simulink model "Plant0"  (R2020b)
settings: Solver=FixedStepAuto  StartTime=0.0  StopTime=5  FixedStep=1e-06  RelTol=1e-3
settings Model: Creator=99714  LastModifiedBy=99714
settings DataIOCC: SaveOutput=off  SaveTime=off

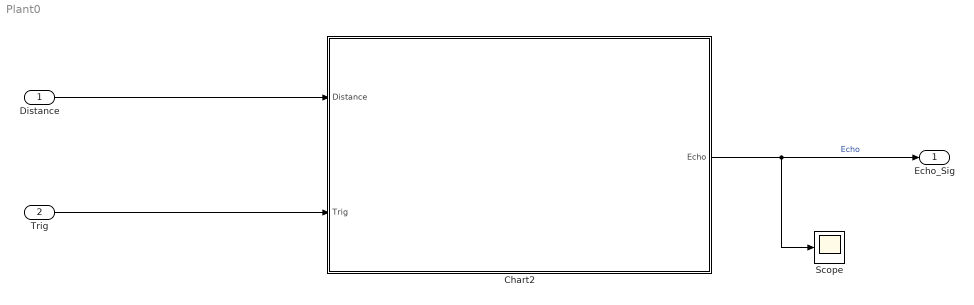
== system Plant0 ==
  Distance : Inport  OutDataTypeStr=single  PortDimensions=1
  Trig : Inport  Port=2  OutDataTypeStr=single  PortDimensions=1
  Chart2 : Stateflow chart  TreatAsAtomicUnit=on
  Scope : Scope
  Echo_Sig : Outport  OutDataTypeStr=single  PortDimensions=1  SampleTime=[9.9999999999999995e-07,0]
  wires:
  Trig/1 -> Chart2/2(Trig)
  Chart2/1(Echo) -> Scope/1, Echo_Sig/1  "Echo"
  Distance/1 -> Chart2/1(Distance)

== stateflow chart Plant0/Chart2 ==
  state Echo_On
    en:
    Echo=1;
    DIS=Distance;
  state Echo_Off
    en:
    Echo=0;
  state On_standby
    en:
    Echo=0
  (default) -> On_standby
  On_standby -> Echo_On : [Trig==1]
  Echo_On -> Echo_Off : after(58*DIS,usec)
  Echo_Off -> On_standby : [Echo==0]
  data: Distance input single; Trig input single; Echo output single; DIS local
